simulink model "test_fuse_data"  (Simulink 7.6)
settings: Solver=ode45  StartTime=0.0  StopTime=100.0  RelTol=1e-3
libraries: simulink x48
settings Model: Creator=jporter  LastModifiedBy=jporter

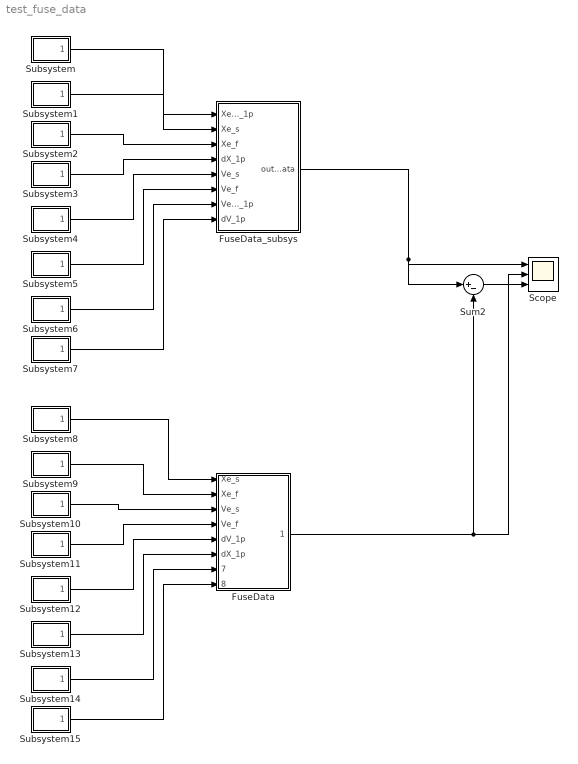
== system test_fuse_data ==
  FuseData : Stateflow chart  TreatAsAtomicUnit=on
  FuseData_subsys : Subsystem
  Scope : Scope  NumInputPorts=3
      settings: YMin=-5~-5~-5  YMax=5~5~5
  Subsystem : Subsystem
  Subsystem1 : Subsystem
  Subsystem10 : Subsystem
  Subsystem11 : Subsystem
  Subsystem12 : Subsystem
  Subsystem13 : Subsystem
  Subsystem14 : Subsystem
  Subsystem15 : Subsystem
  Subsystem2 : Subsystem
  Subsystem3 : Subsystem
  Subsystem4 : Subsystem
  Subsystem5 : Subsystem
  Subsystem6 : Subsystem
  Subsystem7 : Subsystem
  Subsystem8 : Subsystem
  Subsystem9 : Subsystem
  Sum2 : Sum  Inputs=|+-
  wires:
  Subsystem/1(Out1) -> FuseData_subsys/1(Xe_sh_1p)
  Subsystem1/1(Out1) -> FuseData_subsys/2(Xe_s)
  Subsystem2/1(Out1) -> FuseData_subsys/3(Xe_f)
  Subsystem3/1(Out1) -> FuseData_subsys/4(dX_1p)
  Subsystem4/1(Out1) -> FuseData_subsys/5(Ve_s)
  Subsystem5/1(Out1) -> FuseData_subsys/6(Ve_f)
  Subsystem6/1(Out1) -> FuseData_subsys/7(Ve_sh_1p)
  Subsystem7/1(Out1) -> FuseData_subsys/8(dV_1p)
  Subsystem8/1(Out1) -> FuseData/1(Xe_s)
  Subsystem9/1(Out1) -> FuseData/2(Xe_f)
  Subsystem10/1(Out1) -> FuseData/3(Ve_s)
  Subsystem11/1(Out1) -> FuseData/4(Ve_f)
  Subsystem12/1(Out1) -> FuseData/5(dV_1p)
  Subsystem13/1(Out1) -> FuseData/6(dX_1p)
  Subsystem14/1(Out1) -> FuseData/7(Ve_sh_1p)
  Subsystem15/1(Out1) -> FuseData/8(Xe_sh_1p)
  Sum2/1 -> Scope/3
  FuseData_subsys/1(out_data) -> Scope/1, Sum2/1
  FuseData/1(out_data) -> Scope/2, Sum2/2

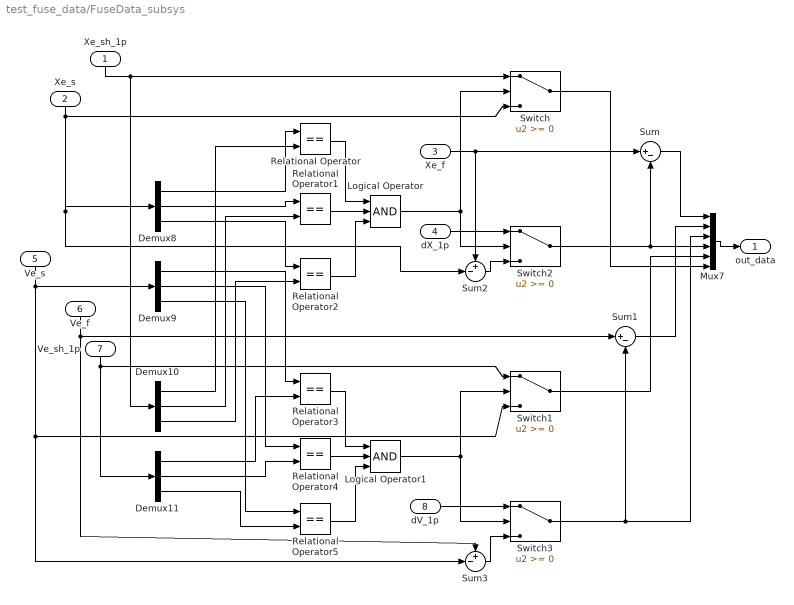
== system test_fuse_data/FuseData_subsys ==
  Xe_sh_1p : Inport
  Xe_s : Inport  Port=2
  Xe_f : Inport  Port=3
  dX_1p : Inport  Port=4
  Ve_s : Inport  Port=5
  Ve_f : Inport  Port=6
  Ve_sh_1p : Inport  Port=7
  dV_1p : Inport  Port=8
  Demux{8..11} (4 alike) : Demux  Outputs=3
  Logical Operator : Logic  Inputs=3  AllPortsSameDT=off  OutDataTypeStr=boolean
  Logical Operator1 : Logic  Inputs=3  AllPortsSameDT=off  OutDataTypeStr=boolean
  Mux7 : Mux  Inputs=6
  Relational Operator{,1..5} (6 alike) : RelationalOperator  Operator===  OutDataTypeStr=boolean
  Sum : Sum  Inputs=|+-
  Sum1 : Sum  Inputs=|+-
  Sum2 : Sum  Inputs=+-|
  Sum3 : Sum  Inputs=+-|
  Switch{,1..3} (4 alike) : Switch
  out_data : Outport
  wires:
  Relational Operator/1 -> Logical Operator/1
  Relational Operator1/1 -> Logical Operator/2
  Relational Operator2/1 -> Logical Operator/3
  Logical Operator/1 -> Switch/2, Switch2/2
  Relational Operator3/1 -> Logical Operator1/1
  Relational Operator4/1 -> Logical Operator1/2
  Relational Operator5/1 -> Logical Operator1/3
  Logical Operator1/1 -> Switch1/2, Switch3/2
  Switch2/1 -> Mux7/4, Sum/2
  Switch/1 -> Mux7/6
  Switch1/1 -> Mux7/5
  Switch3/1 -> Mux7/3, Sum1/2
  Sum/1 -> Mux7/1
  Sum1/1 -> Mux7/2
  Demux8/1 -> Relational Operator/1
  Demux10/1 -> Relational Operator/2
  Demux8/2 -> Relational Operator1/1
  Demux10/2 -> Relational Operator1/2
  Demux8/3 -> Relational Operator2/1
  Demux10/3 -> Relational Operator2/2
  Demux9/1 -> Relational Operator3/1
  Demux9/2 -> Relational Operator4/1
  Demux9/3 -> Relational Operator5/1
  Demux11/1 -> Relational Operator3/2
  Demux11/2 -> Relational Operator4/2
  Demux11/3 -> Relational Operator5/2
  Sum2/1 -> Switch2/3
  Sum3/1 -> Switch3/3
  Xe_sh_1p/1 -> Switch/1, Demux10/1
  Xe_s/1 -> Switch/3, Demux8/1, Sum2/2
  Xe_f/1 -> Sum/1, Sum2/1
  dX_1p/1 -> Switch2/1
  Ve_s/1 -> Switch1/3, Sum3/2, Demux9/1
  Ve_f/1 -> Sum1/1, Sum3/1
  Ve_sh_1p/1 -> Demux11/1, Switch1/1
  dV_1p/1 -> Switch3/1
  Mux7/1 -> out_data/1

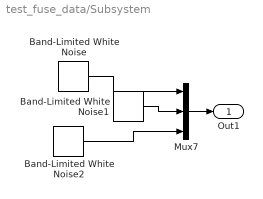
== system test_fuse_data/Subsystem ==
  Band-Limited White Noise : simulink/Sources/Band-Limited White Noise  SystemSampleTime=-1  Cov=0.5  Ts=0.01  seed=[23341]
  Band-Limited White Noise1 : simulink/Sources/Band-Limited White Noise  SystemSampleTime=-1  Cov=0.5  Ts=0.01  seed=[23341]
  Band-Limited White Noise2 : simulink/Sources/Band-Limited White Noise  SystemSampleTime=-1  Cov=0.5  Ts=0.01  seed=[23341]
  Mux7 : Mux  Inputs=3
  Out1 : Outport
  wires:
  Band-Limited White Noise/1 -> Mux7/1
  Band-Limited White Noise1/1 -> Mux7/2
  Band-Limited White Noise2/1 -> Mux7/3
  Mux7/1 -> Out1/1

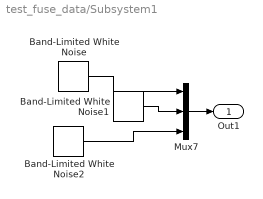
== system test_fuse_data/Subsystem1 ==
  Band-Limited White Noise : simulink/Sources/Band-Limited White Noise  SystemSampleTime=-1  Cov=0.5  Ts=0.01  seed=[23341]
  Band-Limited White Noise1 : simulink/Sources/Band-Limited White Noise  SystemSampleTime=-1  Cov=0.5  Ts=0.01  seed=[23341]
  Band-Limited White Noise2 : simulink/Sources/Band-Limited White Noise  SystemSampleTime=-1  Cov=0.5  Ts=0.01  seed=[23341]
  Mux7 : Mux  Inputs=3
  Out1 : Outport
  wires:
  Band-Limited White Noise/1 -> Mux7/1
  Band-Limited White Noise1/1 -> Mux7/2
  Band-Limited White Noise2/1 -> Mux7/3
  Mux7/1 -> Out1/1

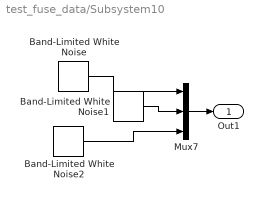
== system test_fuse_data/Subsystem10 ==
  Band-Limited White Noise : simulink/Sources/Band-Limited White Noise  SystemSampleTime=-1  Cov=0.5  Ts=0.01  seed=[23341]
  Band-Limited White Noise1 : simulink/Sources/Band-Limited White Noise  SystemSampleTime=-1  Cov=0.5  Ts=0.01  seed=[23341]
  Band-Limited White Noise2 : simulink/Sources/Band-Limited White Noise  SystemSampleTime=-1  Cov=0.5  Ts=0.01  seed=[23341]
  Mux7 : Mux  Inputs=3
  Out1 : Outport
  wires:
  Band-Limited White Noise/1 -> Mux7/1
  Band-Limited White Noise1/1 -> Mux7/2
  Band-Limited White Noise2/1 -> Mux7/3
  Mux7/1 -> Out1/1

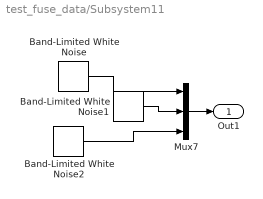
== system test_fuse_data/Subsystem11 ==
  Band-Limited White Noise : simulink/Sources/Band-Limited White Noise  SystemSampleTime=-1  Cov=0.5  Ts=0.01  seed=[23341]
  Band-Limited White Noise1 : simulink/Sources/Band-Limited White Noise  SystemSampleTime=-1  Cov=0.5  Ts=0.01  seed=[23341]
  Band-Limited White Noise2 : simulink/Sources/Band-Limited White Noise  SystemSampleTime=-1  Cov=0.5  Ts=0.01  seed=[23341]
  Mux7 : Mux  Inputs=3
  Out1 : Outport
  wires:
  Band-Limited White Noise/1 -> Mux7/1
  Band-Limited White Noise1/1 -> Mux7/2
  Band-Limited White Noise2/1 -> Mux7/3
  Mux7/1 -> Out1/1

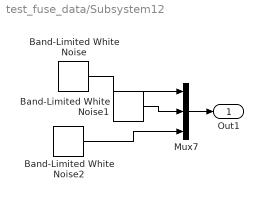
== system test_fuse_data/Subsystem12 ==
  Band-Limited White Noise : simulink/Sources/Band-Limited White Noise  SystemSampleTime=-1  Cov=0.5  Ts=0.01  seed=[23341]
  Band-Limited White Noise1 : simulink/Sources/Band-Limited White Noise  SystemSampleTime=-1  Cov=0.5  Ts=0.01  seed=[23341]
  Band-Limited White Noise2 : simulink/Sources/Band-Limited White Noise  SystemSampleTime=-1  Cov=0.5  Ts=0.01  seed=[23341]
  Mux7 : Mux  Inputs=3
  Out1 : Outport
  wires:
  Band-Limited White Noise/1 -> Mux7/1
  Band-Limited White Noise1/1 -> Mux7/2
  Band-Limited White Noise2/1 -> Mux7/3
  Mux7/1 -> Out1/1

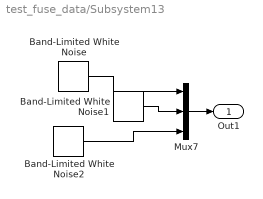
== system test_fuse_data/Subsystem13 ==
  Band-Limited White Noise : simulink/Sources/Band-Limited White Noise  SystemSampleTime=-1  Cov=0.5  Ts=0.01  seed=[23341]
  Band-Limited White Noise1 : simulink/Sources/Band-Limited White Noise  SystemSampleTime=-1  Cov=0.5  Ts=0.01  seed=[23341]
  Band-Limited White Noise2 : simulink/Sources/Band-Limited White Noise  SystemSampleTime=-1  Cov=0.5  Ts=0.01  seed=[23341]
  Mux7 : Mux  Inputs=3
  Out1 : Outport
  wires:
  Band-Limited White Noise/1 -> Mux7/1
  Band-Limited White Noise1/1 -> Mux7/2
  Band-Limited White Noise2/1 -> Mux7/3
  Mux7/1 -> Out1/1

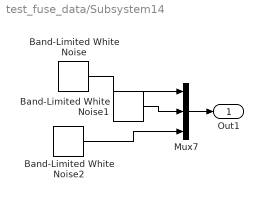
== system test_fuse_data/Subsystem14 ==
  Band-Limited White Noise : simulink/Sources/Band-Limited White Noise  SystemSampleTime=-1  Cov=0.5  Ts=0.01  seed=[23341]
  Band-Limited White Noise1 : simulink/Sources/Band-Limited White Noise  SystemSampleTime=-1  Cov=0.5  Ts=0.01  seed=[23341]
  Band-Limited White Noise2 : simulink/Sources/Band-Limited White Noise  SystemSampleTime=-1  Cov=0.5  Ts=0.01  seed=[23341]
  Mux7 : Mux  Inputs=3
  Out1 : Outport
  wires:
  Band-Limited White Noise/1 -> Mux7/1
  Band-Limited White Noise1/1 -> Mux7/2
  Band-Limited White Noise2/1 -> Mux7/3
  Mux7/1 -> Out1/1

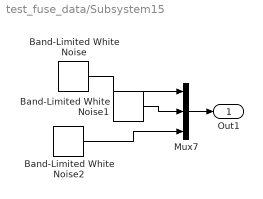
== system test_fuse_data/Subsystem15 ==
  Band-Limited White Noise : simulink/Sources/Band-Limited White Noise  SystemSampleTime=-1  Cov=0.5  Ts=0.01  seed=[23341]
  Band-Limited White Noise1 : simulink/Sources/Band-Limited White Noise  SystemSampleTime=-1  Cov=0.5  Ts=0.01  seed=[23341]
  Band-Limited White Noise2 : simulink/Sources/Band-Limited White Noise  SystemSampleTime=-1  Cov=0.5  Ts=0.01  seed=[23341]
  Mux7 : Mux  Inputs=3
  Out1 : Outport
  wires:
  Band-Limited White Noise/1 -> Mux7/1
  Band-Limited White Noise1/1 -> Mux7/2
  Band-Limited White Noise2/1 -> Mux7/3
  Mux7/1 -> Out1/1

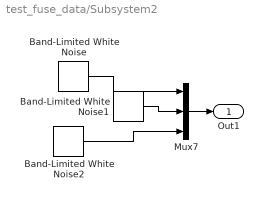
== system test_fuse_data/Subsystem2 ==
  Band-Limited White Noise : simulink/Sources/Band-Limited White Noise  SystemSampleTime=-1  Cov=0.5  Ts=0.01  seed=[23341]
  Band-Limited White Noise1 : simulink/Sources/Band-Limited White Noise  SystemSampleTime=-1  Cov=0.5  Ts=0.01  seed=[23341]
  Band-Limited White Noise2 : simulink/Sources/Band-Limited White Noise  SystemSampleTime=-1  Cov=0.5  Ts=0.01  seed=[23341]
  Mux7 : Mux  Inputs=3
  Out1 : Outport
  wires:
  Band-Limited White Noise/1 -> Mux7/1
  Band-Limited White Noise1/1 -> Mux7/2
  Band-Limited White Noise2/1 -> Mux7/3
  Mux7/1 -> Out1/1

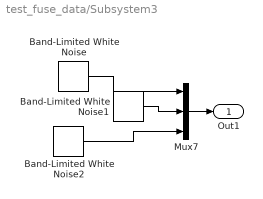
== system test_fuse_data/Subsystem3 ==
  Band-Limited White Noise : simulink/Sources/Band-Limited White Noise  SystemSampleTime=-1  Cov=0.5  Ts=0.01  seed=[23341]
  Band-Limited White Noise1 : simulink/Sources/Band-Limited White Noise  SystemSampleTime=-1  Cov=0.5  Ts=0.01  seed=[23341]
  Band-Limited White Noise2 : simulink/Sources/Band-Limited White Noise  SystemSampleTime=-1  Cov=0.5  Ts=0.01  seed=[23341]
  Mux7 : Mux  Inputs=3
  Out1 : Outport
  wires:
  Band-Limited White Noise/1 -> Mux7/1
  Band-Limited White Noise1/1 -> Mux7/2
  Band-Limited White Noise2/1 -> Mux7/3
  Mux7/1 -> Out1/1

== system test_fuse_data/Subsystem4 ==
  Band-Limited White Noise : simulink/Sources/Band-Limited White Noise  SystemSampleTime=-1  Cov=0.5  Ts=0.01  seed=[23341]
  Band-Limited White Noise1 : simulink/Sources/Band-Limited White Noise  SystemSampleTime=-1  Cov=0.5  Ts=0.01  seed=[23341]
  Band-Limited White Noise2 : simulink/Sources/Band-Limited White Noise  SystemSampleTime=-1  Cov=0.5  Ts=0.01  seed=[23341]
  Mux7 : Mux  Inputs=3
  Out1 : Outport
  wires:
  Band-Limited White Noise/1 -> Mux7/1
  Band-Limited White Noise1/1 -> Mux7/2
  Band-Limited White Noise2/1 -> Mux7/3
  Mux7/1 -> Out1/1

== system test_fuse_data/Subsystem5 ==
  Band-Limited White Noise : simulink/Sources/Band-Limited White Noise  SystemSampleTime=-1  Cov=0.5  Ts=0.01  seed=[23341]
  Band-Limited White Noise1 : simulink/Sources/Band-Limited White Noise  SystemSampleTime=-1  Cov=0.5  Ts=0.01  seed=[23341]
  Band-Limited White Noise2 : simulink/Sources/Band-Limited White Noise  SystemSampleTime=-1  Cov=0.5  Ts=0.01  seed=[23341]
  Mux7 : Mux  Inputs=3
  Out1 : Outport
  wires:
  Band-Limited White Noise/1 -> Mux7/1
  Band-Limited White Noise1/1 -> Mux7/2
  Band-Limited White Noise2/1 -> Mux7/3
  Mux7/1 -> Out1/1

== system test_fuse_data/Subsystem6 ==
  Band-Limited White Noise : simulink/Sources/Band-Limited White Noise  SystemSampleTime=-1  Cov=0.5  Ts=0.01  seed=[23341]
  Band-Limited White Noise1 : simulink/Sources/Band-Limited White Noise  SystemSampleTime=-1  Cov=0.5  Ts=0.01  seed=[23341]
  Band-Limited White Noise2 : simulink/Sources/Band-Limited White Noise  SystemSampleTime=-1  Cov=0.5  Ts=0.01  seed=[23341]
  Mux7 : Mux  Inputs=3
  Out1 : Outport
  wires:
  Band-Limited White Noise/1 -> Mux7/1
  Band-Limited White Noise1/1 -> Mux7/2
  Band-Limited White Noise2/1 -> Mux7/3
  Mux7/1 -> Out1/1

== system test_fuse_data/Subsystem7 ==
  Band-Limited White Noise : simulink/Sources/Band-Limited White Noise  SystemSampleTime=-1  Cov=0.5  Ts=0.01  seed=[23341]
  Band-Limited White Noise1 : simulink/Sources/Band-Limited White Noise  SystemSampleTime=-1  Cov=0.5  Ts=0.01  seed=[23341]
  Band-Limited White Noise2 : simulink/Sources/Band-Limited White Noise  SystemSampleTime=-1  Cov=0.5  Ts=0.01  seed=[23341]
  Mux7 : Mux  Inputs=3
  Out1 : Outport
  wires:
  Band-Limited White Noise/1 -> Mux7/1
  Band-Limited White Noise1/1 -> Mux7/2
  Band-Limited White Noise2/1 -> Mux7/3
  Mux7/1 -> Out1/1

== system test_fuse_data/Subsystem8 ==
  Band-Limited White Noise : simulink/Sources/Band-Limited White Noise  SystemSampleTime=-1  Cov=0.5  Ts=0.01  seed=[23341]
  Band-Limited White Noise1 : simulink/Sources/Band-Limited White Noise  SystemSampleTime=-1  Cov=0.5  Ts=0.01  seed=[23341]
  Band-Limited White Noise2 : simulink/Sources/Band-Limited White Noise  SystemSampleTime=-1  Cov=0.5  Ts=0.01  seed=[23341]
  Mux7 : Mux  Inputs=3
  Out1 : Outport
  wires:
  Band-Limited White Noise/1 -> Mux7/1
  Band-Limited White Noise1/1 -> Mux7/2
  Band-Limited White Noise2/1 -> Mux7/3
  Mux7/1 -> Out1/1

== system test_fuse_data/Subsystem9 ==
  Band-Limited White Noise : simulink/Sources/Band-Limited White Noise  SystemSampleTime=-1  Cov=0.5  Ts=0.01  seed=[23341]
  Band-Limited White Noise1 : simulink/Sources/Band-Limited White Noise  SystemSampleTime=-1  Cov=0.5  Ts=0.01  seed=[23341]
  Band-Limited White Noise2 : simulink/Sources/Band-Limited White Noise  SystemSampleTime=-1  Cov=0.5  Ts=0.01  seed=[23341]
  Mux7 : Mux  Inputs=3
  Out1 : Outport
  wires:
  Band-Limited White Noise/1 -> Mux7/1
  Band-Limited White Noise1/1 -> Mux7/2
  Band-Limited White Noise2/1 -> Mux7/3
  Mux7/1 -> Out1/1

== matlab function FuseData ==
  data: Xe_s input single size=[3]; out_data output single; Xe_f input single size=[3]; Ve_s input single size=[3]; Ve_f input single size=[3]; dV_1p input double; dX_1p input double; Ve_sh_1p input double; Xe_sh_1p input double
function out_data  = fcn(Xe_s, Xe_f, Ve_s, Ve_f,dV_1p,dX_1p,Ve_sh_1p,Xe_sh_1p)
%function [Xe,Ve,dV_1,dX_1,Ve_sh_1,Xe_sh_1] = fcn(Xe_s, Xe_f, Ve_s, Ve_f,dV_1p,dX_1p,Ve_sh_1p,Xe_sh_1p)
%#eml

%persistent dV_1p dX_1p Ve_sh_1p Xe_sh_1p

%if ( isempty( dV_1p ) )
%   dV_1p = zeros(size(Ve_s),'single');
%   dX_1p = zeros(size(Xe_s),'single');
%   Ve_sh_1p = dV_1p;
%   Xe_sh_1p = dX_1p;
%end

if ((Xe_s(1) ~= Xe_sh_1p(1)) || (Xe_s(2) ~= Xe_sh_1p(2)) || (Xe_s(3) ~= Xe_sh_1p(3)))
    Xe_sh_1 = Xe_s;
    dX_1 = Xe_f - Xe_s;
else
    Xe_sh_1 = Xe_sh_1p;
    dX_1 = dX_1p;
end


if ((Ve_s(1) ~= Ve_sh_1p(1)) || (Ve_s(2) ~= Ve_sh_1p(2)) || (Ve_s(3) ~= Ve_sh_1p(3)))
    Ve_sh_1 = Ve_s;
    dV_1 = Ve_f - Ve_s;
else
    Ve_sh_1 = Ve_sh_1p;
    dV_1 = dV_1p;
end

%dV_1p = dV_1;
%dX_1p = dX_1;
%Ve_sh_1p = Ve_sh_1;
%Xe_sh_1p = Xe_sh_1;

Xe = Xe_f - dX_1;
Ve = Ve_f - dV_1;

out_data = [Xe; Ve; dV_1; dX_1; Ve_sh_1; Xe_sh_1 ];
